simulink model "Question3"  (R2023b)
settings: Solver=VariableStepAuto  StartTime=0.0  StopTime=20.0  RelTol=1e-3
values from neighbouring files (symbols this model uses):
  den = cell2mat(HY3_N1_D.denominator)    [Question_3.m]    (also in threeDiskOscillator_RIG_template_2023.m)
  den2 = cell2mat(HY3_N2_D.denominator)    [Question_3.m]    (also in threeDiskOscillator.m; threeDiskOscillator_RIG_template_2023.m)
  num_HU2_N1_D = cell2mat(HU2_N1_D.numerator)    [Question_3.m]    (also in threeDiskOscillator.m; threeDiskOscillator_RIG_template_2023.m)
  num_HY1_N1_D = cell2mat(HY1_N1_D.numerator)    [Question_3.m]    (also in threeDiskOscillator.m; threeDiskOscillator_RIG_template_2023.m)
  num_HY2_N1_D = cell2mat(HY2_N1_D.numerator)    [Question_3.m]    (also in threeDiskOscillator.m; threeDiskOscillator_RIG_template_2023.m)
  num_HY2_N2_D = cell2mat(HY2_N2_D.numerator)    [Question_3.m]    (also in threeDiskOscillator.m; threeDiskOscillator_RIG_template_2023.m)
  num_HY3_N1_D = cell2mat(HY3_N1_D.numerator)    [Question_3.m]    (also in threeDiskOscillator.m; threeDiskOscillator_RIG_template_2023.m)
  num_HY3_N2_D = cell2mat(HY3_N2_D.numerator)    [Question_3.m]    (also in threeDiskOscillator.m; threeDiskOscillator_RIG_template_2023.m)
settings Model: Creator=andre  LastModifiedBy=andre

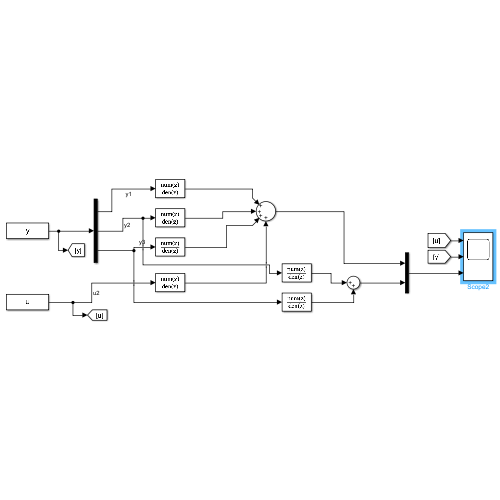
[thumbnail: Simulink's stored preview of the top-level diagram]
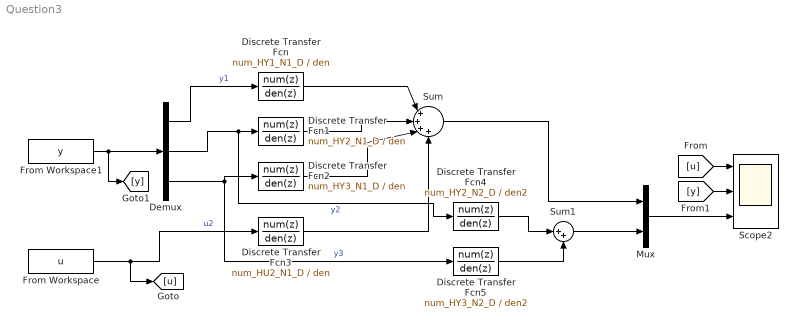
== system Question3 ==
  Demux : Demux  Outputs=3
  Discrete Transfer Fcn : DiscreteTransferFcn  Numerator=num_HY1_N1_D  Denominator=den
  Discrete Transfer Fcn1 : DiscreteTransferFcn  Numerator=num_HY2_N1_D  Denominator=den
  Discrete Transfer Fcn2 : DiscreteTransferFcn  Numerator=num_HY3_N1_D  Denominator=den
  Discrete Transfer Fcn3 : DiscreteTransferFcn  Numerator=num_HU2_N1_D  Denominator=den
  Discrete Transfer Fcn4 : DiscreteTransferFcn  Numerator=num_HY2_N2_D  Denominator=den2
  Discrete Transfer Fcn5 : DiscreteTransferFcn  Numerator=num_HY3_N2_D  Denominator=den2
  From Workspace : FromWorkspace  VariableName=u
  From Workspace1 : FromWorkspace  VariableName=y  SampleTime=0.004
  Mux : Mux  Inputs=2
  Scope2 : Scope  NumInputPorts=3
  Sum : Sum  Inputs=|++++
  Sum1 : Sum  Inputs=|++
  wires:
  Mux/1 -> Scope2/3
  Sum1/1 -> Mux/2
  Demux/1 -> Discrete Transfer Fcn/1  "y1"
  Discrete Transfer Fcn4/1 -> Sum1/1
  Demux/3 -> Discrete Transfer Fcn5/1, Discrete Transfer Fcn2/1  "y3"
  From Workspace/1 -> [u], Discrete Transfer Fcn3/1  "u2"
  Demux/2 -> Discrete Transfer Fcn4/1, Discrete Transfer Fcn1/1  "y2"
  Discrete Transfer Fcn5/1 -> Sum1/2
  Sum/1 -> Mux/1
  Discrete Transfer Fcn3/1 -> Sum/4
  Discrete Transfer Fcn1/1 -> Sum/2
  Discrete Transfer Fcn2/1 -> Sum/3
  Discrete Transfer Fcn/1 -> Sum/1
  From Workspace1/1 -> [y], Demux/1
  [y] -> Scope2/2
  [u] -> Scope2/1
